simulink library "simeventsentitymanage1"  (Simulink 7.0)
undefined symbols (not defined in the file or in its folder): des_support, gcbh
settings Model: Creator=mclune  LastModifiedBy=mramaswa  ExtModeAutoUpdateStatusClock=off

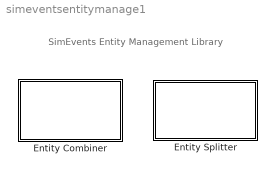
== system simeventsentitymanage1 ==
  note: SimEvents Entity Management Library
  Entity Combiner : Subsystem  Priority=1  LoadFcn=des_support('desLoadFcn',gcbh)  StartFcn=des_support('desStartFcn',gcbh)  StopFcn=des_support('desStopFcn',gcbh)  mask(Entity Combiner){NumberInputPorts=3, RetainComponentEntities=on, AttributeAccessibility=on, TimerAccessibility=on, AttributeCopied=on, TimerCopied=on, StatNumberDeparted=Off, EvaluatedNumPorts=3}
      mask prompts: NumberInputPorts "Number of entity input ports:"; RetainComponentEntities "Retain structure in departing entity"; AttributeAccessibility "Make attributes accessible in departing entity"; TimerAccessibility "Make timers accessible in departing entity"; AttributeCopied "Copy attributes to departing entity"; TimerCopied "Copy timers to departing entity"; StatNumberDeparted "Number of entities departed, #d:"; EvaluatedNumPorts "Evaluated number of ports"
      mask help: Create one new entity for each set of entities arriving simultaneously at all input ports. The departing entity can include information about the structure, attributes, and timers of the arriving entities. Retaining structure makes this block's operation reversible via the Entity Spliter block. Accessibility of attributes or timers requires uniqueness of attribute names or timer tags, respectively, among all arriving entities in the set.
      mask init:
      | des_entitycombinermask(gcb,'init','apply')
      settings: CopyFcn=des_support('desCopyFcn',gcbh)  DeleteFcn=des_support('desDeleteFcn',gcbh)  UndoDeleteFcn=des_support('desUndoDeleteFcn',gcbh)  ModelCloseFcn=des_support('desModelCloseFcn',gcbh)  PreSaveFcn=des_support('desPreSaveFcn',gcbh)  PostSaveFcn=des_support('desPostSaveFcn',gcbh)  NameChangeFcn=des_support('desNameChangeFcn',gcbh)  CloseFcn=des_support('desCloseFcn',gcbh)  ErrorFcn=des_error_redirect
      mask Help: helpview(simeventsbhelp)
      mask StyleString: edit,checkbox,checkbox,checkbox,checkbox,checkbox,popup(Off|On|Upon stop or pause),edit
      mask CallbackString: des_entitycombinermask(gcb,'cbNumberInputPorts','noapply');|des_entitycombinermask(gcb,'cbSpecifyRetainStructure','noapply');|||||des_entitycombinermask(gcb,'cbStatNumberDeparted','noapply');|
      mask TabNameString: Entity Combiner,Entity Combiner,Entity Combiner,Entity Combiner,Entity Combiner,Entity Combiner,Statistics,Statistics
      mask Display:
      | image(des_iconLoad('combinerStruct.jpg'),'center');
      | port_label('LConn',1,'IN1');
      | port_label('LConn',2,'IN2');
      | port_label('LConn',3,'IN3');
      | port_label('RConn',1,'OUT');
  Entity Splitter : Subsystem  Priority=1  LoadFcn=des_support('desLoadFcn',gcbh)  StartFcn=des_support('desStartFcn',gcbh)  StopFcn=des_support('desStopFcn',gcbh)  mask(Entity Splitter){NumberOutputPorts=3, SplitEntityWhen=All entity output ports are not blocked, OutputPortPrecedence=OUT1 port, InitialSeed=56789, ActionUponPortMismatch=Continue, ActionUponBlocking=Discard entity, StatNumberArrived=Off, StatNumberDeparted=Off, EvaluatedNumPorts=3}
      mask prompts: NumberOutputPorts "Number of entity output ports:"; SplitEntityWhen "Split entity when:"; OutputPortPrecedence "Departure port precedence:"; InitialSeed "Initial seed:"; ActionUponPortMismatch "If number of component entities does not match number of entity output ports:"; ActionUponBlocking "If an output port becomes blocked during split:"; StatNumberArrived "Number of entities arrived, #a:"; StatNumberDeparted "Number of entities departed, #d:"; EvaluatedNumPorts "Evaluated number of ports"
      mask help:
      | Divide a composite entity into its components and output the component entities through each entity output port that is not blocked. A composite entity is the output of the Entity Combiner block when retaining structure.
      |
      | This block accepts an entity to split only when the availabilities of the subsequent blocks' entity input ports meet the criteria listed in the 'Split entity when' parameter.
      mask init:
      | des_entitysplittermask(gcb,'init','apply')
      settings: CopyFcn=des_support('desCopyFcn',gcbh)  DeleteFcn=des_support('desDeleteFcn',gcbh)  UndoDeleteFcn=des_support('desUndoDeleteFcn',gcbh)  ModelCloseFcn=des_support('desModelCloseFcn',gcbh)  PreSaveFcn=des_support('desPreSaveFcn',gcbh)  PostSaveFcn=des_support('desPostSaveFcn',gcbh)  NameChangeFcn=des_support('desNameChangeFcn',gcbh)  CloseFcn=des_support('desCloseFcn',gcbh)  ErrorFcn=des_error_redirect
      mask Help: helpview(simeventsbhelp)
      mask StyleString: edit,popup(All entity output ports are not blocked|Any entity output port is not blocked),popup(OUT1 port|Round robin|Equiprobable),edit,popup(Continue|Warn and continue|Error),popup(Discard entity|Warn and discard entity|Error),popup(Off|On|Upon stop or pause),popup(Off|On|Upon stop or pause),edit
      mask CallbackString: des_entitysplittermask(gcb,'cbNumberOutputPorts','noapply');|des_entitysplittermask(gcb,'cbSplitEntityWhen','noapply');|des_entitysplittermask(gcb,'cbPortPrecedence','noapply');|des_entitysplittermask(gcb,'cbInitialSeed','noapply');||des_entitysplittermask(gcb,'cbActionUponBlocking','noapply');|des_entitysplittermask(gcb,'cbStatNumberArrived','noapply');|des_entitysplittermask(gcb,'cbStatNumberDeparted','noapply');|
      mask TabNameString: Splitter,Splitter,Splitter,Splitter,Splitter,Splitter,Statistics,Statistics,Statistics
      mask Display:
      | image(des_iconLoad('entitySplitter.jpg'),'center');
      | port_label('LConn',1,'IN');
      | port_label('RConn',1,'OUT1');
      | port_label('RConn',2,'OUT2');
      | port_label('RConn',3,'OUT3');

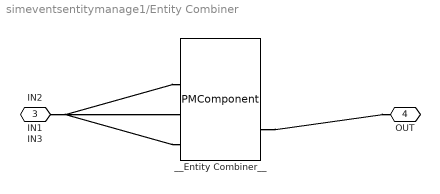
== system simeventsentitymanage1/Entity Combiner ==
  __Entity Combiner__ : PMComponent  PhysicalDomain=simevents  SubClassName=DES_SUBENTITYCOMBINER  LeftPortType=desPortIn  RightPortType=desPortOut  IconImage=body_q.bmp  LConnTagsString=DI|DI|DI|DI  RConnTagsString=DO|DO
      mask Display:
      | port_label('LConn',1,'p');
      | port_label('LConn',2,'IN1');
      | port_label('LConn',3,'IN2');
      | port_label('LConn',4,'IN3');
      | port_label('RConn',1,'#d');
      | port_label('RConn',2,'OUT');
  IN1 : PMIOPort  Port=1  Side=Left
  IN2 : PMIOPort  Port=2  Side=Left
  IN3 : PMIOPort  Port=3  Side=Left
  OUT : PMIOPort  Orientation=left  Port=4  Side=Right
  connections:
  IN1/RConn1 -- __Entity Combiner__/LConn2
  IN2/RConn1 -- __Entity Combiner__/LConn3
  IN3/RConn1 -- __Entity Combiner__/LConn4
  __Entity Combiner__/RConn2 -- OUT/RConn1

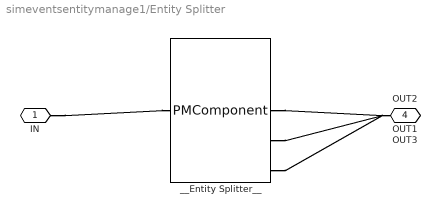
== system simeventsentitymanage1/Entity Splitter ==
  __Entity Splitter__ : PMComponent  PhysicalDomain=simevents  SubClassName=DES_SPLITTER_ALL  LeftPortType=desPortIn  RightPortType=desPortOut  LConnTagsString=DI  RConnTagsString=DO|DO|DO|DO|DO
      mask Display:
      | port_label('LConn',1,'IN');
      | port_label('RConn',1,'#a');
      | port_label('RConn',2,'#d');
      | port_label('RConn',3,'OUT1');
      | port_label('RConn',4,'OUT2');
      | port_label('RConn',5,'OUT3');
  IN : PMIOPort  Port=1  Side=Left
  OUT1 : PMIOPort  Orientation=left  Port=2  Side=Right
  OUT2 : PMIOPort  Orientation=left  Port=3  Side=Right
  OUT3 : PMIOPort  Orientation=left  Port=4  Side=Right
  connections:
  IN/RConn1 -- __Entity Splitter__/LConn1
  __Entity Splitter__/RConn3 -- OUT1/RConn1
  __Entity Splitter__/RConn4 -- OUT2/RConn1
  __Entity Splitter__/RConn5 -- OUT3/RConn1
